simulink model "untitled"  (R2013a)
settings: Solver=ode45  StartTime=0.0  StopTime=10.0  RelTol=1e-3
settings Model: Creator=pkushal  LastModifiedBy=pkushal

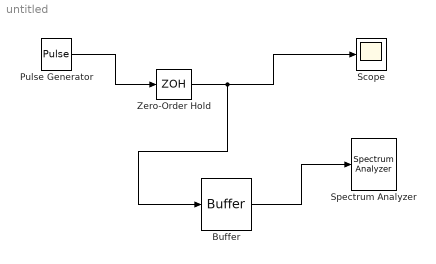
== system untitled ==
  Buffer : Buffer  N=1024  TreatMby1Signals=One channel
  Pulse Generator : DiscretePulseGenerator
  Scope : Scope
  Spectrum Analyzer : SpectrumAnalyzer
      settings: CopyFcn=scopeextensions.ScopeBlock.callback(gcbh, 'onBlockCopy', gcbh);  DeleteFcn=scopeextensions.ScopeBlock.callback(gcbh, 'onBlockDelete');  PreSaveFcn=scopeextensions.ScopeBlock.callback(gcbh, 'onModelSave');  NameChangeFcn=scopeextensions.ScopeBlock.callback(gcbh, 'onBlockRename');  CloseFcn=scopeextensions.ScopeBlock.callback(gcbh, 'onBlockClose');  PreDeleteFcn=scopeextensions.ScopeBlock.callback(gcbh, 'onBlockPreDelete');
  Zero-Order Hold : ZeroOrderHold
  wires:
  Pulse Generator/1 -> Zero-Order Hold/1
  Zero-Order Hold/1 -> Buffer/1, Scope/1
  Buffer/1 -> Spectrum Analyzer/1
